simulink model "disturbance_rejection_example"  (R2017a)
settings: Solver=VariableStepAuto  StartTime=0.0  StopTime=30  RelTol=1e-3
settings Model: Creator=GusBus  LastModifiedBy=GusBus

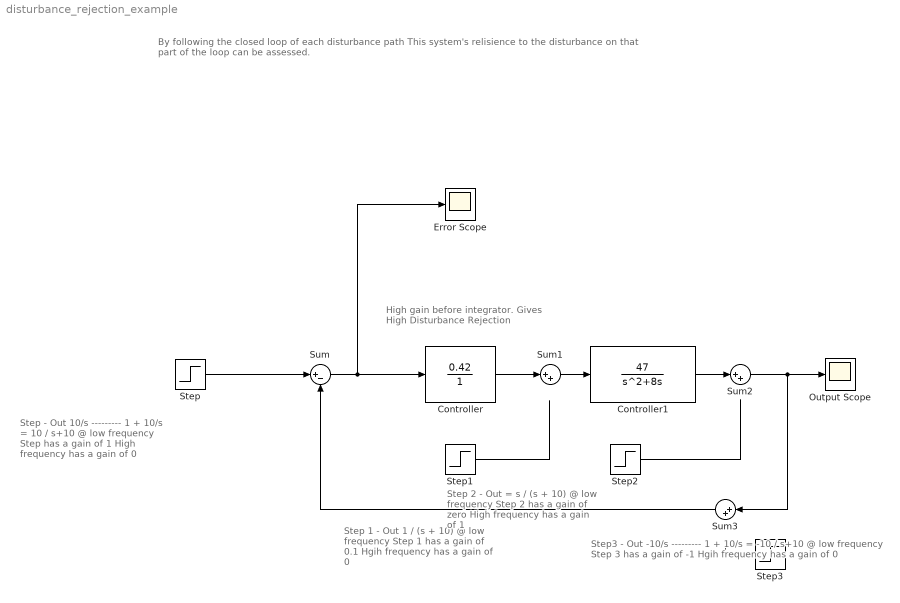
== system disturbance_rejection_example ==
  note: By following the closed loop of each disturbance path
      | This system's relisience to the disturbance on that part of the loop
      | can be assessed.
  note: Step - Out
      | 10/s
      | ---------
      | 1 + 10/s
      |
      | = 10 / s+10
      |
      | @ low frequency Step
      | has a gain of 1
      | High frequency has a gain of 0
  note: High gain before integrator.
      | Gives High Disturbance Rejection
  note: Step 1 - Out
      |
      | 1 / (s + 10)
      |
      | @ low frequency Step
      | 1 has a gain of 0.1
      | Hgih frequency has a gain of 0
  note: Step 2 - Out
      | = s / (s + 10)
      |
      | @ low frequency Step
      | 2 has a gain of zero
      | High frequency has a gain of 1
  note: Step3 - Out
      | -10/s
      | ---------
      | 1 + 10/s
      |
      | = -10 / s+10
      |
      | @ low frequency Step
      | 3 has a gain of -1
      | Hgih frequency has a gain of 0
  Controller : TransferFcn  Numerator=[0.42]  Denominator=[1]
  Controller1 : TransferFcn  Numerator=[47]  Denominator=[1 8 0]
  Error Scope : Scope
  Output Scope : Scope
  Step : Step  Time=0.1  SampleTime=0
  Step1 : Step  Time=2  SampleTime=0
  Step2 : Step  Time=3  SampleTime=0
  Step3 : Step  Time=5  SampleTime=0
  Sum : Sum  Inputs=|+-
  Sum1 : Sum  Inputs=|++
  Sum2 : Sum  Inputs=|++
  Sum3 : Sum  Inputs=|++
  wires:
  Controller/1 -> Sum1/1
  Sum/1 -> Error Scope/1, Controller/1
  Step/1 -> Sum/1
  Sum2/1 -> Sum3/1, Output Scope/1
  Sum1/1 -> Controller1/1
  Controller1/1 -> Sum2/1
  Step2/1 -> ?
  Step1/1 -> ?
  Sum3/1 -> Sum/2
  Step3/1 -> ?
